simulink model "pH_control_loops"  (R2024b)
settings: Solver=ode45  StartTime=0.0  StopTime=900  RelTol=1e-3
values from neighbouring files (symbols this model uses):
  pH_const = struct()    [prepare_sim.m]
undefined symbols (not defined in the file or in its folder): sigbuilder_block
settings Model: Creator=User  LastModifiedBy=HP
settings SolverCC: AlgebraicLoopSolver=TrustRegion
settings DebuggingCC: UnconnectedInputMsg=warning  UnconnectedOutputMsg=warning  UnconnectedLineMsg=warning  ArithmeticOperatorsInVariantConditions=warning
settings ModelReferenceCC: EnableRefExpFcnMdlSchedulingChecks=on
settings SFSimCC: CustomCodeUndefinedFunction=UseInterfaceOnly
settings RTWCC: GPUComputeCapability=3.5

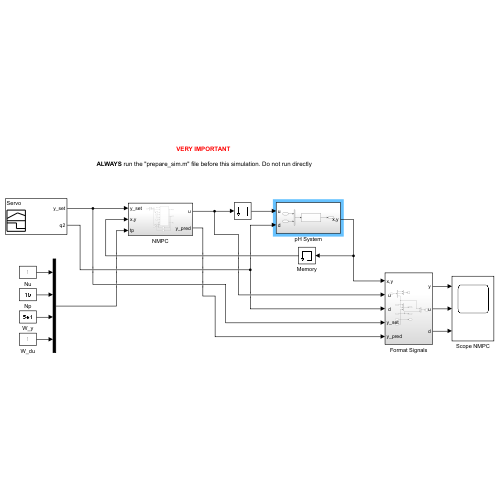
[thumbnail: Simulink's stored preview of the top-level diagram]
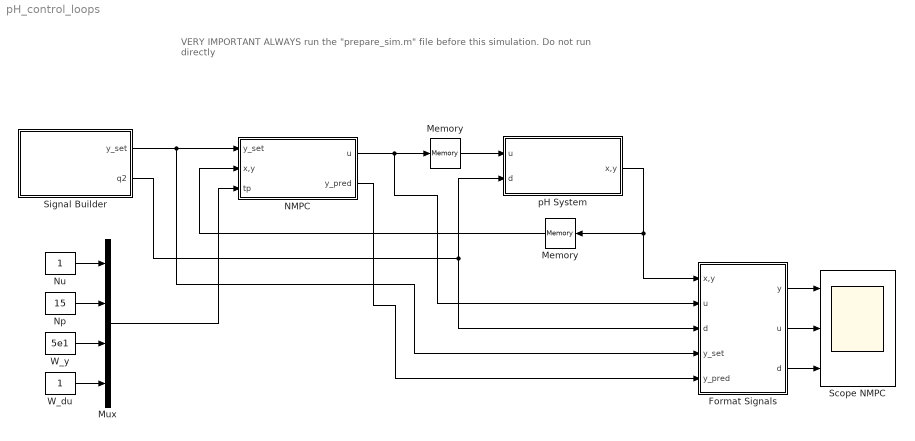
== system pH_control_loops ==
  note: VERY IMPORTANT
      |
      | ALWAYS run the "prepare_sim.m" file before this simulation. Do not run directly
  " Memory " : Memory  InitialCondition=[pH_const.x_0(1); pH_const.x_0(2); pH_const.y_0(1)]
  Format Signals : Subsystem
  Memory : Memory  InitialCondition=pH_const.u_0
  Mux : Mux
  NMPC : Subsystem
  Np : Constant  Value=15
  Nu : Constant
  Scope NMPC : Scope  NumInputPorts=3
  Signal Builder : Subsystem  Tag=STV Subsys  LoadFcn=sigbuilder_block('load');  StartFcn=sigbuilder_block('start');  StopFcn=sigbuilder_block('stop');  ClipboardFcn=sigbuilder_block('clipboard');  mask(Sigbuilder block){tuvar=[0:10]}
      mask help: Simulink:masks:SigbuilderBlock_MD
      mask init:
      | if ~strcmp(get_param(bdroot(gcbh),'SimulationStatus'),'stopped') tuvar = sigbuilder_block('maskInit'); end
      settings: CopyFcn=sigbuilder_block('copy');  DeleteFcn=sigbuilder_block('delete');  ModelCloseFcn=sigbuilder_block('modelClose');  PreSaveFcn=sigbuilder_block('preSave');  PauseFcn=sigbuilder_block('pause');  ContinueFcn=sigbuilder_block('continue');  NameChangeFcn=sigbuilder_block('namechange');  OpenFcn=sigbuilder_block('open',[184.5 249 640.5 331.5 ]);  CloseFcn=sigbuilder_block('close');
      mask Display: plot(0, 0, 100, 100,[2, 2, 32, 32, 2], [68, 8, 8, 68, 68],[32, 2], [38, 38], [32, 19, 2],[53, 60, 44], [32, 17, 17, 2],[16, 16, 31, 31]);txt = getActiveGroup(gcbh);text(2, 100, txt,'verticalAlignment', 'top');
  W_du : Constant
  W_y : Constant  Value=5e1
  pH System : Subsystem
  wires:
  W_du/1 -> Mux/4
  Memory/1 -> pH System/1(u)
  W_y/1 -> Mux/3
  NMPC/1(u) -> Memory/1, Format Signals/2(" u ")
  Np/1 -> Mux/2
  Signal Builder/2(q2) -> pH System/2(d), Format Signals/3(" d ")
  pH System/1(x,y) -> " Memory "/1, Format Signals/1(x,y)
  Signal Builder/1(y_set) -> NMPC/1(y_set), Format Signals/4(y_set)
  Format Signals/2(u) -> Scope NMPC/2
  Nu/1 -> Mux/1
  Format Signals/3(d) -> Scope NMPC/3
  Format Signals/1(y) -> Scope NMPC/1
  Mux/1 -> NMPC/3(tp)
  " Memory "/1 -> NMPC/2(x,y)
  NMPC/2(y_pred) -> Format Signals/5(y_pred)

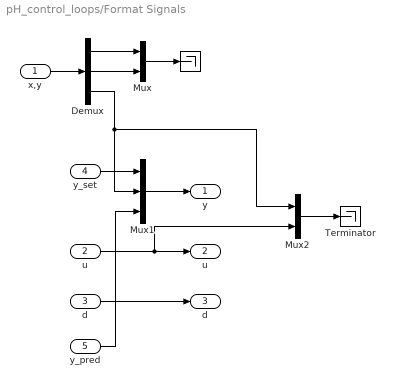
== system pH_control_loops/Format Signals ==
  x,y : Inport
  " u " : Inport  Port=2
  " d " : Inport  Port=3
  y_set : Inport  Port=4
  y_pred : Inport  Port=5
  "  " : Terminator
  Demux : Demux  Outputs=3
  Mux : Mux  Inputs=2
  Mux1 : Mux  Inputs=3
  Mux2 : Mux  Inputs=2
  Terminator : Terminator
  y : Outport  VectorParamsAs1DForOutWhenUnconnected=off
  u : Outport  Port=2  VectorParamsAs1DForOutWhenUnconnected=off
  d : Outport  Port=3  VectorParamsAs1DForOutWhenUnconnected=off
  wires:
  x,y/1 -> Demux/1
  Demux/3 -> Mux1/2, Mux2/1
  Demux/2 -> Mux/2
  Demux/1 -> Mux/1
  Mux/1 -> "  "/1
  y_set/1 -> Mux1/1
  " u "/1 -> Mux2/2, u/1
  Mux1/1 -> y/1
  " d "/1 -> d/1
  Mux2/1 -> Terminator/1
  y_pred/1 -> Mux1/3

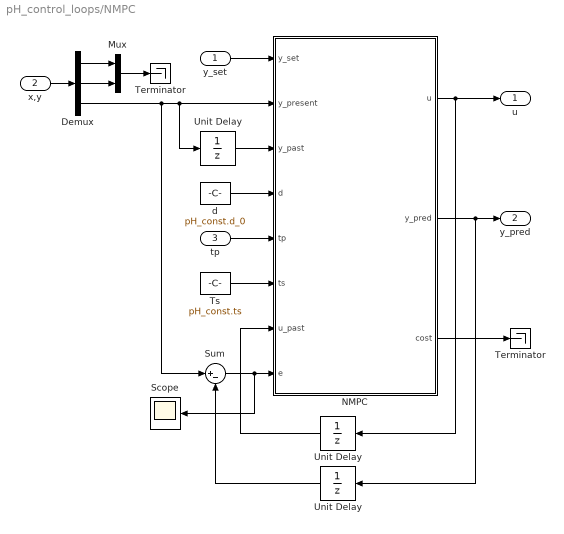
== system pH_control_loops/NMPC ==
  y_set : Inport
  x,y : Inport  Port=2
  tp : Inport  Port=3
  "  Unit Delay  " : UnitDelay  InitialCondition=pH_const.y_0  SampleTime=pH_const.ts  HasFrameUpgradeWarning=on
  " Unit Delay " : UnitDelay  InitialCondition=pH_const.y_0  SampleTime=pH_const.ts  HasFrameUpgradeWarning=on
  Demux : Demux  Outputs=3
  Mux : Mux  Inputs=2
  "NMPC " : MATLAB Function  TreatAsAtomicUnit=on  SystemSampleTime=pH_const.ts
  Scope : Scope
  Sum : Sum  Inputs=|+-
  Terminator : Terminator
  "Terminator " : Terminator
  Ts : Constant  Value=pH_const.ts
  Unit Delay : UnitDelay  InitialCondition=pH_const.u_0  SampleTime=pH_const.ts  HasFrameUpgradeWarning=on
  d : Constant  Value=pH_const.d_0
  u : Outport  VectorParamsAs1DForOutWhenUnconnected=off
  y_pred : Outport  Port=2  VectorParamsAs1DForOutWhenUnconnected=off
  wires:
  "NMPC "/1(u) -> u/1, Unit Delay/1
  Unit Delay/1 -> "NMPC "/7(u_past)
  y_set/1 -> "NMPC "/1(y_set)
  tp/1 -> "NMPC "/5(tp)
  d/1 -> "NMPC "/4(d)
  Ts/1 -> "NMPC "/6(ts)
  "NMPC "/3(cost) -> "Terminator "/1
  Demux/3 -> Sum/1, " Unit Delay "/1, "NMPC "/2(y_present)
  " Unit Delay "/1 -> "NMPC "/3(y_past)
  x,y/1 -> Demux/1
  Demux/2 -> Mux/2
  Demux/1 -> Mux/1
  Mux/1 -> Terminator/1
  "NMPC "/2(y_pred) -> y_pred/1, "  Unit Delay  "/1
  "  Unit Delay  "/1 -> Sum/2
  Sum/1 -> "NMPC "/8(e), Scope/1

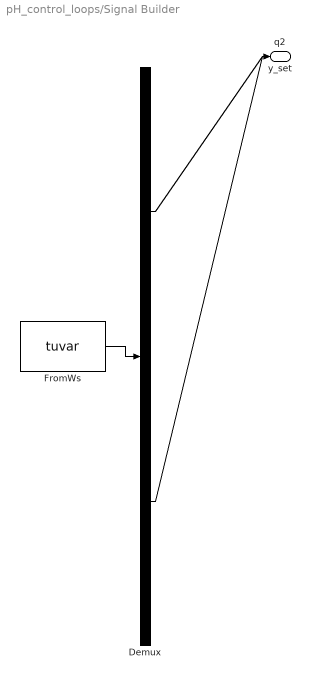
== system pH_control_loops/Signal Builder ==
  Demux : Demux  Tag=STV Demux  Outputs=2
      settings: DisplayOption=none
  FromWs : FromWorkspace  Tag=STV FromWs  VariableName=tuvar
      SigBuilderData=|
      | common.afterFinalStr = 'Extrapolate'
      | common.sampleTime = 0
      | dataSet(1).timeRange = [0 1200]
      | dataSet(1).name = 'Servo'
      | dataSet(2).timeRange = [0 600]
      | dataSet(2).name = 'Regulatory'
      | sbobj.Groups(1).Name = 'Servo'
      | sbobj.Groups(1).Signals(1).Name = 'y_set'
      | sbobj.Groups(1).Signals(1).XData = [0 400 400 800 800 900 1200]
      | sbobj.Groups(1).Signals(1).YData = [9 9 5 5 7 7 7]
      | sbobj.Groups(1).Signals(2).Name = 'q2'
      | sbobj.Groups(1).Signals(2).XData = [0 1200]
      | sbobj.Groups(1).Signals(2).YData = [0.55 0.55]
      | sbobj.Groups(1).TimeRange = [0 1200]
      | sbobj.Groups(2).Name = 'Regulatory'
      | sbobj.Groups(2).Signals(1).Name = 'y_set'
      | sbobj.Groups(2).Signals(1).XData = [0 600]
      | sbobj.Groups(2).Signals(1).YData = [7 7]
      | sbobj.Groups(2).Signals(2).Name = 'q2'
      | sbobj.Groups(2).Signals(2).XData = [0 150 150 300 300 450 450 600]
      | sbobj.Groups(2).Signals(2).YData = [1.5 1.5 0.25 0.25 2 2 0.55 0.55]
      | sbobj.Groups(2).TimeRange = [0 600]
  y_set : Outport  Tag=STV Outport  VectorParamsAs1DForOutWhenUnconnected=off
  q2 : Outport  Tag=STV Outport  Port=2  VectorParamsAs1DForOutWhenUnconnected=off
  wires:
  FromWs/1 -> Demux/1
  Demux/1 -> y_set/1
  Demux/2 -> q2/1

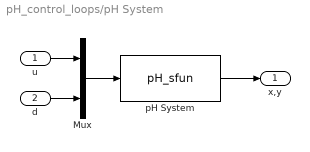
== system pH_control_loops/pH System ==
  u : Inport
  d : Inport  Port=2
  Mux : Mux  Inputs=2
  pH System : S-Function  FunctionName=pH_sfun  SFunctionDeploymentMode=off  EnableBusSupport=off
  x,y : Outport  VectorParamsAs1DForOutWhenUnconnected=off
  wires:
  u/1 -> Mux/1
  d/1 -> Mux/2
  Mux/1 -> pH System/1
  pH System/1 -> x,y/1

== matlab function pH_control_loops/NMPC/NMPC  ==
  data: u output size=[1,1]; y_pred output; cost output size=[1,1]; y_set input; y_present input; y_past input; d input; tp input; ts input; u_past input; e input
function [u, y_pred, cost] = nmpc(y_set,y_present,y_past,d,tp,ts,u_past,e)
    u = u_past; cost = 0; y_pred = y_present;
    coder.extrinsic('get_control_input');
    [u, y_pred, cost] = get_control_input(y_set,y_present,y_past,u_past,d,tp,ts,e,1);
end
